simulink model "CP_model"  (R2015a)
settings: Solver=ode45  StartTime=0.0  StopTime=6  RelTol=1e-3
libraries: simulink x3
settings Model: Creator=root  LastModifiedBy=root

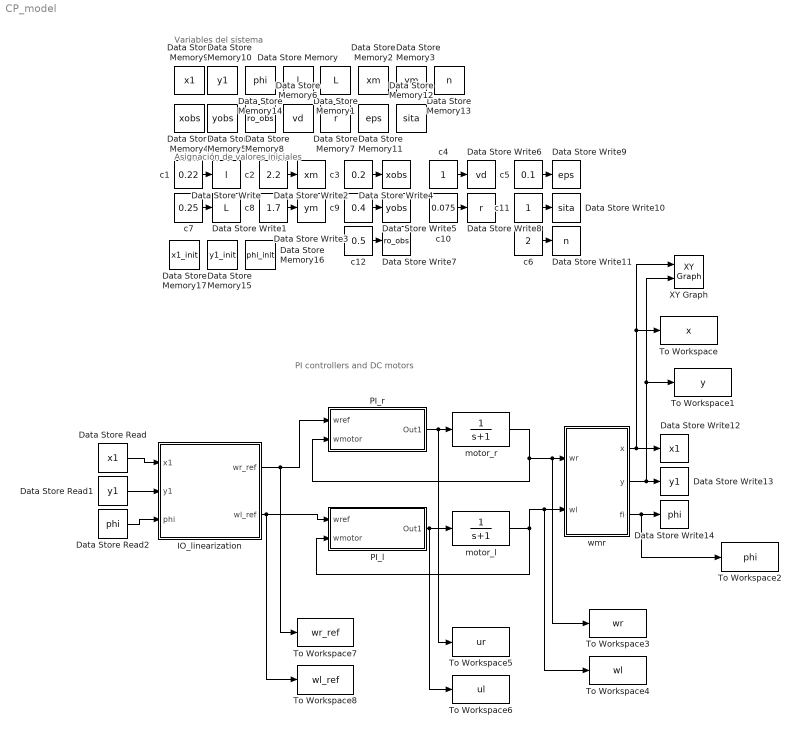
== system CP_model ==
  note: PI controllers and DC motors
  note: Variables del sistema
  note: Asignación de valores iniciales
  Data Store Memory : DataStoreMemory  DataStoreName=l  ReadBeforeWriteMsg=warning  WriteAfterWriteMsg=warning  WriteAfterReadMsg=warning
  Data Store Memory1 : DataStoreMemory  DataStoreName=L  ReadBeforeWriteMsg=warning  WriteAfterWriteMsg=warning  WriteAfterReadMsg=warning
  Data Store Memory10 : DataStoreMemory  DataStoreName=y1  ReadBeforeWriteMsg=warning  WriteAfterWriteMsg=warning  WriteAfterReadMsg=warning
  Data Store Memory11 : DataStoreMemory  DataStoreName=eps  ReadBeforeWriteMsg=warning  WriteAfterWriteMsg=warning  WriteAfterReadMsg=warning
  Data Store Memory12 : DataStoreMemory  DataStoreName=sita  ReadBeforeWriteMsg=warning  WriteAfterWriteMsg=warning  WriteAfterReadMsg=warning
  Data Store Memory13 : DataStoreMemory  DataStoreName=n  ReadBeforeWriteMsg=warning  WriteAfterWriteMsg=warning  WriteAfterReadMsg=warning
  Data Store Memory14 : DataStoreMemory  DataStoreName=phi  ReadBeforeWriteMsg=warning  WriteAfterWriteMsg=warning  WriteAfterReadMsg=warning
  Data Store Memory15 : DataStoreMemory  DataStoreName=y1_init  ReadBeforeWriteMsg=warning  WriteAfterWriteMsg=warning  WriteAfterReadMsg=warning
  Data Store Memory16 : DataStoreMemory  DataStoreName=phi_init  ReadBeforeWriteMsg=warning  WriteAfterWriteMsg=warning  WriteAfterReadMsg=warning
  Data Store Memory17 : DataStoreMemory  DataStoreName=x1_init  ReadBeforeWriteMsg=warning  WriteAfterWriteMsg=warning  WriteAfterReadMsg=warning
  Data Store Memory2 : DataStoreMemory  DataStoreName=xm  ReadBeforeWriteMsg=warning  WriteAfterWriteMsg=warning  WriteAfterReadMsg=warning
  Data Store Memory3 : DataStoreMemory  DataStoreName=ym  ReadBeforeWriteMsg=warning  WriteAfterWriteMsg=warning  WriteAfterReadMsg=warning
  Data Store Memory4 : DataStoreMemory  DataStoreName=xobs  ReadBeforeWriteMsg=warning  WriteAfterWriteMsg=warning  WriteAfterReadMsg=warning
  Data Store Memory5 : DataStoreMemory  DataStoreName=yobs  ReadBeforeWriteMsg=warning  WriteAfterWriteMsg=warning  WriteAfterReadMsg=warning
  Data Store Memory6 : DataStoreMemory  DataStoreName=vd  ReadBeforeWriteMsg=warning  WriteAfterWriteMsg=warning  WriteAfterReadMsg=warning
  Data Store Memory7 : DataStoreMemory  DataStoreName=r  ReadBeforeWriteMsg=warning  WriteAfterWriteMsg=warning  WriteAfterReadMsg=warning
  Data Store Memory8 : DataStoreMemory  DataStoreName=ro_obs  ReadBeforeWriteMsg=warning  WriteAfterWriteMsg=warning  WriteAfterReadMsg=warning
  Data Store Memory9 : DataStoreMemory  DataStoreName=x1  ReadBeforeWriteMsg=warning  WriteAfterWriteMsg=warning  WriteAfterReadMsg=warning
  Data Store Read : DataStoreRead  DataStoreName=x1
  Data Store Read1 : DataStoreRead  DataStoreName=y1
  Data Store Read2 : DataStoreRead  DataStoreName=phi
  Data Store Write : DataStoreWrite  DataStoreName=l
  Data Store Write1 : DataStoreWrite  DataStoreName=L
  Data Store Write10 : DataStoreWrite  DataStoreName=sita
  Data Store Write11 : DataStoreWrite  DataStoreName=n
  Data Store Write12 : DataStoreWrite  DataStoreName=x1
  Data Store Write13 : DataStoreWrite  DataStoreName=y1
  Data Store Write14 : DataStoreWrite  DataStoreName=phi
  Data Store Write2 : DataStoreWrite  DataStoreName=xm
  Data Store Write3 : DataStoreWrite  DataStoreName=ym
  Data Store Write4 : DataStoreWrite  DataStoreName=xobs
  Data Store Write5 : DataStoreWrite  DataStoreName=yobs
  Data Store Write6 : DataStoreWrite  DataStoreName=vd
  Data Store Write7 : DataStoreWrite  DataStoreName=ro_obs
  Data Store Write8 : DataStoreWrite  DataStoreName=r
  Data Store Write9 : DataStoreWrite  DataStoreName=eps
  IO_linearization : Subsystem
  PI_l : Subsystem
  PI_r : Subsystem
  To Workspace : ToWorkspace  VariableName=x  SaveFormat=Timeseries  SampleTime=-1
  To Workspace1 : ToWorkspace  VariableName=y  SaveFormat=Timeseries  SampleTime=-1
  To Workspace2 : ToWorkspace  VariableName=phi  SaveFormat=Timeseries  SampleTime=-1
  To Workspace3 : ToWorkspace  VariableName=wr  SaveFormat=Timeseries  SampleTime=-1
  To Workspace4 : ToWorkspace  VariableName=wl  SaveFormat=Timeseries  SampleTime=-1
  To Workspace5 : ToWorkspace  VariableName=ur  SaveFormat=Timeseries  SampleTime=-1
  To Workspace6 : ToWorkspace  VariableName=ul  SaveFormat=Timeseries  SampleTime=-1
  To Workspace7 : ToWorkspace  VariableName=wr_ref  SaveFormat=Timeseries  SampleTime=-1
  To Workspace8 : ToWorkspace  VariableName=wl_ref  SaveFormat=Timeseries  SampleTime=-1
  XY Graph : simulink/Sinks/XY Graph  xmin=-1  xmax=1  ymin=-1  ymax=1  st=-1
  "c1 " : Constant  Value=0.22
  c10 : Constant  Value=0.075
  c11 : Constant
  c12 : Constant  Value=0.5
  c2 : Constant  Value=2.2
  c3 : Constant  Value=0.2
  c4 : Constant
  c5 : Constant  Value=0.1
  c6 : Constant  Value=2
  c7 : Constant  Value=0.25
  c8 : Constant  Value=1.7
  c9 : Constant  Value=0.4
  motor_l : TransferFcn  Denominator=[1 1]
  motor_r : TransferFcn  Denominator=[1 1]
  wmr : Subsystem
  wires:
  "c1 "/1 -> Data Store Write/1
  c7/1 -> Data Store Write1/1
  c2/1 -> Data Store Write2/1
  c8/1 -> Data Store Write3/1
  c3/1 -> Data Store Write4/1
  c9/1 -> Data Store Write5/1
  c12/1 -> Data Store Write7/1
  c4/1 -> Data Store Write6/1
  c10/1 -> Data Store Write8/1
  c5/1 -> Data Store Write9/1
  c11/1 -> Data Store Write10/1
  c6/1 -> Data Store Write11/1
  Data Store Read/1 -> IO_linearization/1(x1)
  Data Store Read1/1 -> IO_linearization/2(y1)
  Data Store Read2/1 -> IO_linearization/3(phi)
  PI_r/1(Out1) -> To Workspace5/1, motor_r/1
  PI_l/1(Out1) -> To Workspace6/1, motor_l/1
  motor_l/1 -> PI_l/2(wmotor), To Workspace4/1, wmr/2(wl)
  IO_linearization/2(wl_ref) -> To Workspace8/1, PI_l/1(wref)
  wmr/2(y) -> XY Graph/2, To Workspace1/1, Data Store Write13/1
  wmr/1(x) -> XY Graph/1, To Workspace/1, Data Store Write12/1
  wmr/3(fi) -> To Workspace2/1, Data Store Write14/1
  IO_linearization/1(wr_ref) -> To Workspace7/1, PI_r/1(wref)
  motor_r/1 -> PI_r/2(wmotor), To Workspace3/1, wmr/1(wr)

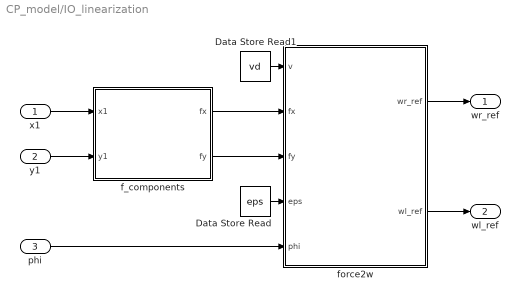
== system CP_model/IO_linearization ==
  x1 : Inport
  y1 : Inport  Port=2
  phi : Inport  Port=3
  Data Store Read : DataStoreRead  DataStoreName=eps
  Data Store Read1 : DataStoreRead  DataStoreName=vd
  f_components : Subsystem
  force2w : Subsystem
  wr_ref : Outport
  wl_ref : Outport  Port=2
  wires:
  f_components/1(fx) -> force2w/2(fx)
  f_components/2(fy) -> force2w/3(fy)
  force2w/1(wr_ref) -> wr_ref/1
  force2w/2(wl_ref) -> wl_ref/1
  x1/1 -> f_components/1(x1)
  y1/1 -> f_components/2(y1)
  phi/1 -> force2w/5(phi)
  Data Store Read/1 -> force2w/4(eps)
  Data Store Read1/1 -> force2w/1("v ")

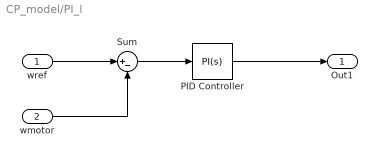
== system CP_model/PI_l ==
  wref : Inport
  wmotor : Inport  Port=2
  PID Controller : simulink/Continuous/PID Controller  Controller=PI  TimeDomain=Continuous-time  SampleTime=-1  IntegratorMethod=Forward Euler  FilterMethod=Forward Euler  Form=Parallel  UseFilter=on  ControllerParametersSource=internal  P=7  I=16  D=0  N=100  InitialConditionSource=internal  InitialConditionForIntegrator=0  InitialConditionForFilter=0  ExternalReset=none  LimitOutput=off  UpperSaturationLimit=inf  LowerSaturationLimit=-inf  LinearizeAsGain=on  AntiWindupMode=none  Kb=1  TrackingMode=off  Kt=1  PParamMin=[]  PParamMax=[]  IParamMin=[]  IParamMax=[]  DParamMin=[]  DParamMax=[]  NParamMin=[]  NParamMax=[]  KbParamMin=[]  KbParamMax=[]  KtParamMin=[]  KtParamMax=[]  POutMin=[]  POutMax=[]  IOutMin=[]  IOutMax=[]  DOutMin=[]  DOutMax=[]  NOutMin=[]  NOutMax=[]  KbOutMin=[]  KbOutMax=[]  KtOutMin=[]  KtOutMax=[]  IntegratorOutMin=[]  IntegratorOutMax=[]  FilterOutMin=[]  FilterOutMax=[]  SumOutMin=[]  SumOutMax=[]  SumI1OutMin=[]  SumI1OutMax=[]  SumI2OutMin=[]  SumI2OutMax=[]  SumI3OutMin=[]  SumI3OutMax=[]  SumDOutMin=[]  SumDOutMax=[]  SaturationOutMin=[]  SaturationOutMax=[]  IntegratorContinuousStateAttributes=''  IntegratorStateMustResolveToSignalObject=off  IntegratorRTWStateStorageClass=Auto  FilterContinuousStateAttributes=''  FilterStateMustResolveToSignalObject=off  FilterRTWStateStorageClass=Auto  DifferentiatorICPrevScaledInput=0  DifferentiatorOutMin=[]  DifferentiatorOutMax=[]
  Sum : Sum  Inputs=|+-
  Out1 : Outport
  wires:
  Sum/1 -> PID Controller/1
  wref/1 -> Sum/1
  wmotor/1 -> Sum/2
  PID Controller/1 -> Out1/1

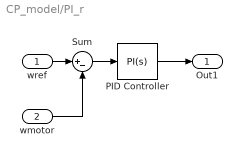
== system CP_model/PI_r ==
  wref : Inport
  wmotor : Inport  Port=2
  PID Controller : simulink/Continuous/PID Controller  Controller=PI  TimeDomain=Continuous-time  SampleTime=-1  IntegratorMethod=Forward Euler  FilterMethod=Forward Euler  Form=Parallel  UseFilter=on  ControllerParametersSource=internal  P=7  I=16  D=0  N=100  InitialConditionSource=internal  InitialConditionForIntegrator=0  InitialConditionForFilter=0  ExternalReset=none  LimitOutput=off  UpperSaturationLimit=inf  LowerSaturationLimit=-inf  LinearizeAsGain=on  AntiWindupMode=none  Kb=1  TrackingMode=off  Kt=1  PParamMin=[]  PParamMax=[]  IParamMin=[]  IParamMax=[]  DParamMin=[]  DParamMax=[]  NParamMin=[]  NParamMax=[]  KbParamMin=[]  KbParamMax=[]  KtParamMin=[]  KtParamMax=[]  POutMin=[]  POutMax=[]  IOutMin=[]  IOutMax=[]  DOutMin=[]  DOutMax=[]  NOutMin=[]  NOutMax=[]  KbOutMin=[]  KbOutMax=[]  KtOutMin=[]  KtOutMax=[]  IntegratorOutMin=[]  IntegratorOutMax=[]  FilterOutMin=[]  FilterOutMax=[]  SumOutMin=[]  SumOutMax=[]  SumI1OutMin=[]  SumI1OutMax=[]  SumI2OutMin=[]  SumI2OutMax=[]  SumI3OutMin=[]  SumI3OutMax=[]  SumDOutMin=[]  SumDOutMax=[]  SaturationOutMin=[]  SaturationOutMax=[]  IntegratorContinuousStateAttributes=''  IntegratorStateMustResolveToSignalObject=off  IntegratorRTWStateStorageClass=Auto  FilterContinuousStateAttributes=''  FilterStateMustResolveToSignalObject=off  FilterRTWStateStorageClass=Auto  DifferentiatorICPrevScaledInput=0  DifferentiatorOutMin=[]  DifferentiatorOutMax=[]
  Sum : Sum  Inputs=|+-
  Out1 : Outport
  wires:
  Sum/1 -> PID Controller/1
  wref/1 -> Sum/1
  wmotor/1 -> Sum/2
  PID Controller/1 -> Out1/1

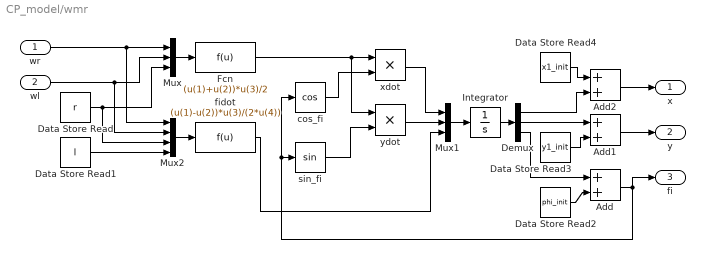
== system CP_model/wmr ==
  wr : Inport
  wl : Inport  Port=2
  Add : Sum
  Add1 : Sum
  Add2 : Sum
  Data Store Read : DataStoreRead  DataStoreName=r
  Data Store Read1 : DataStoreRead  DataStoreName=l
  Data Store Read2 : DataStoreRead  DataStoreName=phi_init
  Data Store Read3 : DataStoreRead  DataStoreName=y1_init
  Data Store Read4 : DataStoreRead  DataStoreName=x1_init
  Demux : Demux  Outputs=3
  Fcn : Fcn  Expr=(u(1)+u(2))*u(3)/2
  Integrator : Integrator
  Mux : Mux  Inputs=3
  Mux1 : Mux  Inputs=3
  Mux2 : Mux
  "cos_fi " : Trigonometry  Operator=cos
  fidot : Fcn  Expr=(u(1)-u(2))*u(3)/(2*u(4))
  "sin_fi " : Trigonometry
  xdot : Product
  ydot : Product
  x : Outport
  y : Outport  Port=2
  fi : Outport  Port=3
  wires:
  wr/1 -> Mux2/1, Mux/1
  wl/1 -> Mux2/2, Mux/2
  Mux/1 -> Fcn/1
  Mux1/1 -> Integrator/1
  Integrator/1 -> Demux/1
  Fcn/1 -> xdot/1, ydot/1
  "cos_fi "/1 -> xdot/2
  xdot/1 -> Mux1/1
  "sin_fi "/1 -> ydot/2
  Data Store Read/1 -> Mux2/3, Mux/3
  ydot/1 -> Mux1/2
  Mux2/1 -> fidot/1
  fidot/1 -> Mux1/3
  Data Store Read1/1 -> Mux2/4
  Demux/3 -> Add/1
  Data Store Read2/1 -> Add/2
  Add/1 -> fi/1, "cos_fi "/1, "sin_fi "/1
  Add1/1 -> y/1
  Data Store Read3/1 -> Add1/2
  Demux/2 -> Add1/1
  Demux/1 -> Add2/2
  Data Store Read4/1 -> Add2/1
  Add2/1 -> x/1

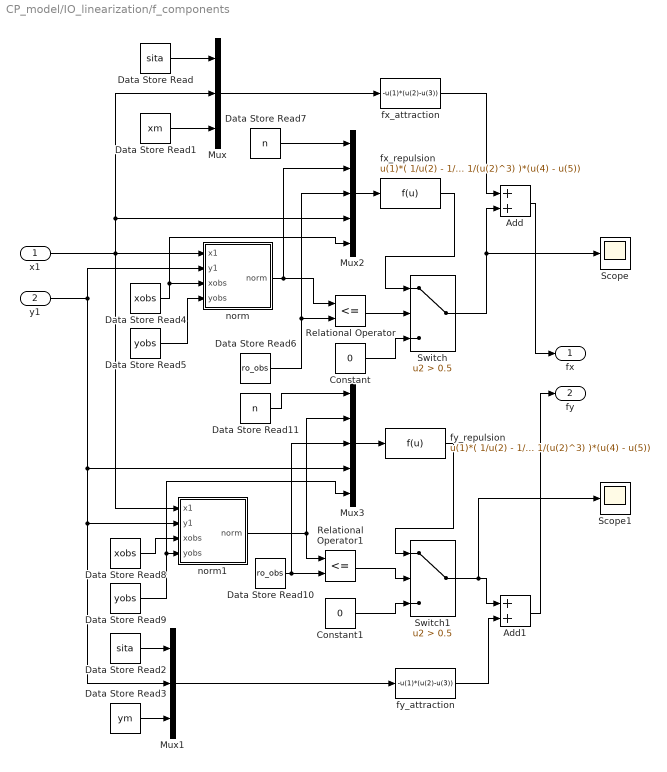
== system CP_model/IO_linearization/f_components ==
  x1 : Inport
  y1 : Inport  Port=2
  Add : Sum
  Add1 : Sum
  Constant : Constant  Value=0
  Constant1 : Constant  Value=0
  Data Store Read : DataStoreRead  DataStoreName=sita
  Data Store Read1 : DataStoreRead  DataStoreName=xm
  Data Store Read10 : DataStoreRead  DataStoreName=ro_obs
  Data Store Read11 : DataStoreRead  DataStoreName=n
  Data Store Read2 : DataStoreRead  DataStoreName=sita
  Data Store Read3 : DataStoreRead  DataStoreName=ym
  Data Store Read4 : DataStoreRead  DataStoreName=xobs
  Data Store Read5 : DataStoreRead  DataStoreName=yobs
  Data Store Read6 : DataStoreRead  DataStoreName=ro_obs
  Data Store Read7 : DataStoreRead  DataStoreName=n
  Data Store Read8 : DataStoreRead  DataStoreName=xobs
  Data Store Read9 : DataStoreRead  DataStoreName=yobs
  Mux : Mux  Inputs=3
  Mux1 : Mux  Inputs=3
  Mux2 : Mux  Inputs=5
  Mux3 : Mux  Inputs=5
  Relational Operator : RelationalOperator  Operator=<=  OutDataTypeStr=boolean
  Relational Operator1 : RelationalOperator  Operator=<=  OutDataTypeStr=boolean
  Scope : Scope
  Scope1 : Scope
  Switch : Switch  Criteria=u2 > Threshold  Threshold=0.5
  Switch1 : Switch  Criteria=u2 > Threshold  Threshold=0.5
  fx_attraction : Fcn  Expr=-u(1)*(u(2)-u(3))
  fx_repulsion : Fcn  Expr=u(1)*( 1/u(2) - 1/u(3) )*( 1/(u(2)^3) )*(u(4) - u(5))
  fy_attraction : Fcn  Expr=-u(1)*(u(2)-u(3))
  fy_repulsion : Fcn  Expr=u(1)*( 1/u(2) - 1/u(3) )*( 1/(u(2)^3) )*(u(4) - u(5))
  norm : Subsystem
  norm1 : Subsystem
  fx : Outport
  fy : Outport  Port=2
  wires:
  fx_attraction/1 -> Add/1
  Data Store Read/1 -> Mux/1
  Data Store Read1/1 -> Mux/3
  Mux/1 -> fx_attraction/1
  Data Store Read2/1 -> Mux1/1
  Data Store Read3/1 -> Mux1/3
  y1/1 -> Mux1/2, norm1/2(y1), Mux3/4, norm/2(y1)
  Mux1/1 -> fy_attraction/1
  Add/1 -> fx/1
  Data Store Read4/1 -> norm/3(xobs), Mux2/5
  Data Store Read5/1 -> norm/4(yobs)
  Relational Operator/1 -> Switch/2
  norm/1(norm) -> Relational Operator/1, Mux2/2
  Data Store Read6/1 -> Relational Operator/2, Mux2/3
  Constant/1 -> Switch/3
  Data Store Read7/1 -> Mux2/1
  x1/1 -> Mux2/4, Mux/2, norm/1(x1), norm1/1(x1)
  Mux2/1 -> fx_repulsion/1
  fx_repulsion/1 -> Switch/1
  Switch/1 -> Scope/1, Add/2
  Data Store Read8/1 -> norm1/3(xobs)
  Data Store Read9/1 -> Mux3/5, norm1/4(yobs)
  Relational Operator1/1 -> Switch1/2
  norm1/1(norm) -> Relational Operator1/1, Mux3/2
  Data Store Read10/1 -> Relational Operator1/2, Mux3/3
  Constant1/1 -> Switch1/3
  Data Store Read11/1 -> Mux3/1
  Mux3/1 -> fy_repulsion/1
  fy_repulsion/1 -> Switch1/1
  Switch1/1 -> Scope1/1, Add1/1
  fy_attraction/1 -> Add1/2
  Add1/1 -> fy/1

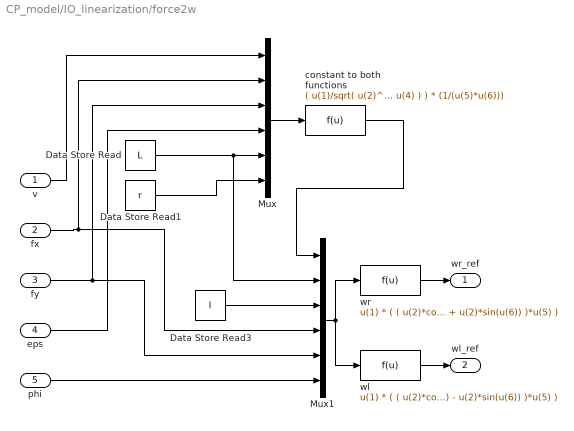
== system CP_model/IO_linearization/force2w ==
  "v " : Inport
  fx : Inport  Port=2
  fy : Inport  Port=3
  eps : Inport  Port=4
  phi : Inport  Port=5
  Data Store Read : DataStoreRead  DataStoreName=L
  Data Store Read1 : DataStoreRead  DataStoreName=r
  Data Store Read3 : DataStoreRead  DataStoreName=l
  Mux : Mux  Inputs=6
  Mux1 : Mux  Inputs=6
  constant to both functions : Fcn  Expr=( u(1)/sqrt( u(2)^2 + u(3)^2 + u(4) ) ) * (1/(u(5)*u(6)))
  wl : Fcn  Expr=u(1) * ( ( u(2)*cos(u(6)) + u(3)*sin(u(6)) )*u(4) - ( u(3)*cos(u(6)) - u(2)*sin(u(6)) )*u(5) )
  wr : Fcn  Expr=u(1) * ( ( u(2)*cos(u(6)) - u(3)*sin(u(6)) )*u(4) + ( u(3)*cos(u(6)) + u(2)*sin(u(6)) )*u(5) )
  wr_ref : Outport
  wl_ref : Outport  Port=2
  wires:
  Mux/1 -> constant to both functions/1
  "v "/1 -> Mux/1
  fx/1 -> Mux1/4, Mux/2
  fy/1 -> Mux1/5, Mux/3
  eps/1 -> Mux/4
  Data Store Read/1 -> Mux/5, Mux1/2
  Data Store Read1/1 -> Mux/6
  constant to both functions/1 -> Mux1/1
  Data Store Read3/1 -> Mux1/3
  phi/1 -> Mux1/6
  wr/1 -> wr_ref/1
  wl/1 -> wl_ref/1
  Mux1/1 -> wl/1, wr/1

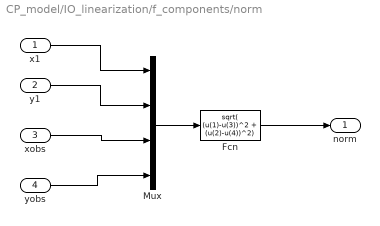
== system CP_model/IO_linearization/f_components/norm ==
  x1 : Inport
  y1 : Inport  Port=2
  xobs : Inport  Port=3
  yobs : Inport  Port=4
  Fcn : Fcn  Expr=sqrt( (u(1)-u(3))^2 + (u(2)-u(4))^2)
  Mux : Mux
  norm : Outport
  wires:
  x1/1 -> Mux/1
  y1/1 -> Mux/2
  xobs/1 -> Mux/3
  yobs/1 -> Mux/4
  Mux/1 -> Fcn/1
  Fcn/1 -> norm/1

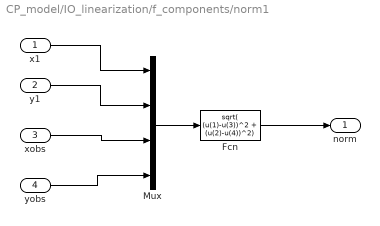
== system CP_model/IO_linearization/f_components/norm1 ==
  x1 : Inport
  y1 : Inport  Port=2
  xobs : Inport  Port=3
  yobs : Inport  Port=4
  Fcn : Fcn  Expr=sqrt( (u(1)-u(3))^2 + (u(2)-u(4))^2)
  Mux : Mux
  norm : Outport
  wires:
  x1/1 -> Mux/1
  y1/1 -> Mux/2
  xobs/1 -> Mux/3
  yobs/1 -> Mux/4
  Mux/1 -> Fcn/1
  Fcn/1 -> norm/1
